simulink model "wheel_loader_dynamic"  (Simulink 8.3)
settings: Solver=ode45  StartTime=0.0  StopTime=8  RelTol=1e-3
values from neighbouring files (symbols this model uses):
  A_cylinder = pi * (r_pis^2 - r_rod^2)    [runSimLoader.m]
  c_fri_1 = 0.7196    [runSimLoader.m]
  c_fri_2 = -.01414    (= -0.01414)    [runSimLoader.m]
  c_fri_3 = 0.3590    (= 0.359)    [runSimLoader.m]
  c_p = 3e4    (= 30000)    [runSimLoader.m]
  c_p_m = [c_p1,c_p2,c_p3,c_p4]    [runSimLoader.m]
  c_r = 0.03    [runSimLoader.m]
  c_t1 = 38.5857    [runSimLoader.m]
  c_t2 = -0.6869    [runSimLoader.m]
  D_pump = 220/1900    (= 0.115789473684)    [runSimLoader.m]
  eta_gb = 0.9    [runSimLoader.m]
  eta_ig = 0.3623    [runSimLoader.m]
  eta_lift = 0.9    [runSimLoader.m]
  eta_vol_eng = 0.9    [runSimLoader.m]
  eta_volumetric = 0.98    [runSimLoader.m]
  gear_ratio = [-60 0 60]    [runSimLoader.m]
  I_ice = 3    [runSimLoader.m]
  k_theta = (diff(r .* sin(theta .* pi ./ 180)) ./ delta_theta)./ (div_delta_L)    [K_theta.m]
  M_boom = 5000    [runSimLoader.m]
  M_buc = 10000    [runSimLoader.m]
  M_load = 10000    [runSimLoader.m]
  M_veh = 32000    [runSimLoader.m]
  M_wheels = 4 .* J_w ./ r_w.^2    [runSimLoader.m]
  n_cyl = 6    [runSimLoader.m]
  n_cyl_hydra = 2    [runSimLoader.m]
  q_hv = 42.9e6    (= 42900000)    [runSimLoader.m]
  r = 2.9    [runSimLoader.m]
  r1 = 1.7    [runSimLoader.m]
  r_w = 0.7    [runSimLoader.m]
  Ra = 287    [runSimLoader.m]
  T_amb = 21 + 273.15    (= 294.15)    [runSimLoader.m]
  theta = -40:0.01:80    [runSimLoader.m]
  theta_1 = (atan((r1 * sin(theta .* pi ./ 180) - yc) ./ (r1 * cos(theta .* pi ./ 180 ) - xc))).* 180 ./ pi    [K_theta.m]
  u_str_max = 1 .* 180 ./ pi    [runSimLoader.m]
  u_str_min = -1 .* 180 ./ pi    [runSimLoader.m]
  Vd = 13e-3    (= 0.013)    [runSimLoader.m]
undefined symbols (not defined in the file or in its folder): sigbuilder_block
settings Model: Creator=beichuan  LastModifiedBy=beichuan
settings SolverCC: ZeroCrossControl=EnableAll
settings DataIOCC: SignalLoggingSaveFormat=Dataset
settings DebuggingCC: UnderspecifiedInitializationDetection=Simplified  MergeDetectMultiDrivingBlocksExec=error  FrameProcessingCompatibilityMsg=error  StateNameClashWarn=none
settings GRTTargetCC: CombineOutputUpdateFcns=on  GRTInterface=off

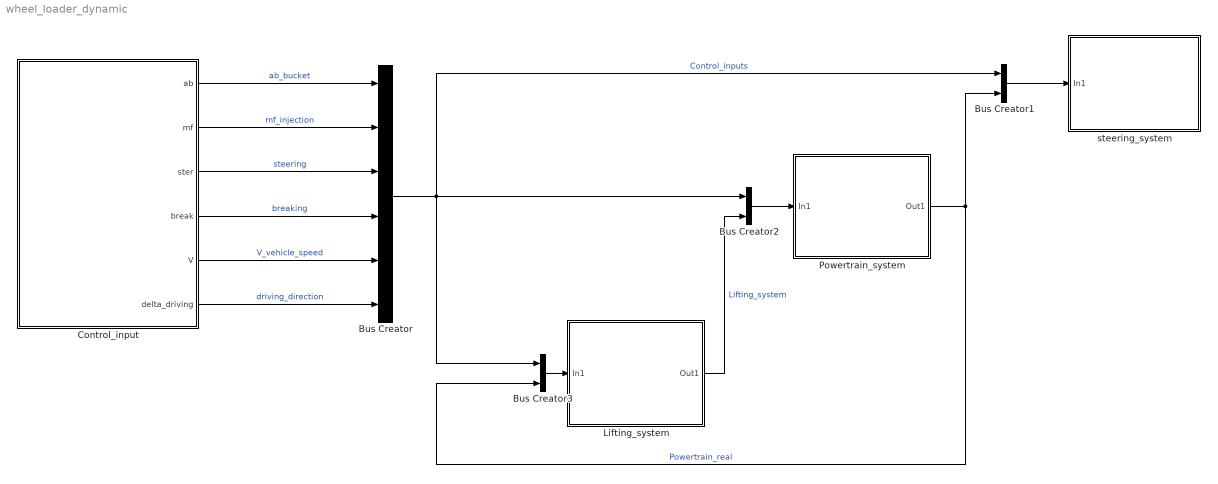
== system wheel_loader_dynamic ==
  Bus Creator : BusCreator  Inputs=6
  Bus Creator1 : BusCreator  Inputs=2
  Bus Creator2 : BusCreator  Inputs=2
  Bus Creator3 : BusCreator  Inputs=2
  Control_input : Subsystem  Tag=STV Subsys  LoadFcn=sigbuilder_block('load');  StartFcn=sigbuilder_block('start');  StopFcn=sigbuilder_block('stop');  ClipboardFcn=sigbuilder_block('clipboard');  mask(Sigbuilder block){}
      mask help: Simulink:masks:SigbuilderBlock_MD
      mask init:
      | if ~strcmp(get_param(bdroot(gcbh),'SimulationStatus'),'stopped') tuvar = sigbuilder_block('maskInit'); end
      settings: CopyFcn=sigbuilder_block('copy');  DeleteFcn=sigbuilder_block('delete');  ModelCloseFcn=sigbuilder_block('modelClose');  PreSaveFcn=sigbuilder_block('preSave');  PauseFcn=sigbuilder_block('pause');  ContinueFcn=sigbuilder_block('continue');  NameChangeFcn=sigbuilder_block('namechange');  OpenFcn=sigbuilder_block('open',[437.6 199.2 550.4 400 ]);  CloseFcn=sigbuilder_block('close');
      mask Display: plot(0, 0, 100, 100,[2, 2, 32, 32, 2], [68, 8, 8, 68, 68],[32, 2], [38, 38], [32, 19, 2],[53, 60, 44], [32, 17, 17, 2],[16, 16, 31, 31]);txt = getActiveGroup(gcbh);text(2, 100, txt,'verticalAlignment', 'top');
  Lifting_system : Subsystem
  Powertrain_system : Subsystem
  steering_system : Subsystem
  wires:
  Control_input/1(ab) -> Bus Creator/1  "ab_bucket"
  Control_input/2(mf) -> Bus Creator/2  "mf_injection"
  Control_input/3(ster) -> Bus Creator/3  "steering"
  Control_input/4(break) -> Bus Creator/4  "breaking"
  Control_input/5(V) -> Bus Creator/5  "V_vehicle_speed"
  Control_input/6(delta_driving) -> Bus Creator/6  "driving_direction"
  Bus Creator/1 -> Bus Creator3/1, Bus Creator2/1, Bus Creator1/1  "Control_inputs"
  Bus Creator1/1 -> steering_system/1(In1)
  Powertrain_system/1(Out1) -> Bus Creator3/2, Bus Creator1/2  "Powertrain_real"
  Lifting_system/1(Out1) -> Bus Creator2/2  "Lifting_system"
  Bus Creator2/1 -> Powertrain_system/1(In1)
  Bus Creator3/1 -> Lifting_system/1(In1)

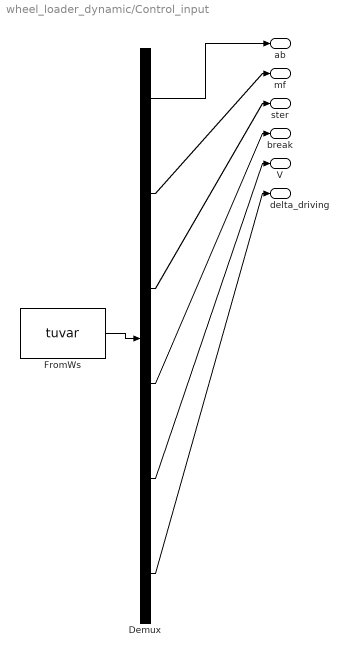
== system wheel_loader_dynamic/Control_input ==
  Demux : Demux  Tag=STV Demux  Outputs=6
  FromWs : FromWorkspace  Tag=STV FromWs  VariableName=tuvar  SampleTime=0  SigBuilderData=DataTag0  VnvData=DataTag1
      SigBuilderData=|
      | common.afterFinalStr = 'Extrapolate'
      | common.sampleTime = 0
      | dataSet.timeRange = [0 8]
      | dataSet.name = 'group1'
      | sbobj.Name = 'Signal Builder'
      | sbobj.Groups.Name = 'group1'
      | sbobj.Groups.Signals(1).Name = 'ab'
      | sbobj.Groups.Signals(1).XData = [0 0.1 0.2 0.3 0.4 0.5 0.6 0.7 0.8 0.9 1 1.1 1.2 1.3 1.4 1.5 1.6 1.7 1.8 1.9 2 2.1 2.2 2.3 2.4 2.5 2.6 2.7 2.8 2.9 3 3.1 3.2 3.3 3.4 3.5 3.6 3.7 3.8 3.9 4 4.1 4.2 4.3 4.4 4.5 4.6 4.7 4.8 4.9 5 5.1 5.2 5.3 5.4 5.5 5.6 5.7 5.8 5.9 6 6.1 6.2 6.3 6.4 6.5 6.6 6.7 6.8 6.9 7 7.1 7.2 7.3 7.4 7.5 7.6 7.7 7.8 7.9 8]
      | sbobj.Groups.Signals(1).YData = [0 0 0 0 0 0 0 0 0 0 0 0.0012 0.0037985136251 0.0308285163776 0.0706953932387 0.351412056152 0.609083402147 0.848224607762 0.935236522355 0.961161574456 0.976823561795 1.00066061107 1.05029294955 1.16939168731 1.3671345995 1.58238370493 1.60753096614 1.49205615194 1.22774566474 0.752127718139 0.227910817506 -0.265290393614 -0.852958987063 -1.50396366639 -1.99154968346 -2.30764290302 -2.40733278282 -2.35080282595 -2.09305807872 -1.59889898156 -0.765384210538 -0.178218185155 -0.0915606936416 -0.0498100743187 -0.0346820809249 -0.0338122763556 -0.0317240113772 -0.0277967834533 -0.0166096496402 -0.00100192678228 0.0428516377649 0.140379851363 0.450867052023 0.779741260666 1.05258935944 1.09202449766 1.07244701349 0.938356729975 0.756165703276 0.614958121977 0.461833195706 0.341701073493 0.326029911001 0.432832369942 0.61853014038 0.839187081384 0.934037985136 0.929967362668 0.763336085879 0.427250206441 -0.0169556840077 -0.531048720066 -0.987943848059 -1.42752546105 -1.83297550234 -2.02650701899 -2.04653637948 -1.88664097624 -1.6395045417 -1.08716396 -0.0666829688749]
      | sbobj.Groups.Signals(2).Name = 'mf'
      | sbobj.Groups.Signals(2).XData = [0 0.1 0.2 0.3 0.4 0.5 0.6 0.7 0.8 0.9 1 1.1 1.2 1.3 1.4 1.5 1.6 1.7 1.8 1.9 2 2.1 2.2 2.3 2.4 2.5 2.6 2.7 2.8 2.9 3 3.1 3.2 3.3 3.4 3.5 3.6 3.7 3.8 3.9 4 4.1 4.2 4.3 4.4 4.5 4.6 4.7 4.8 4.9 5 5.1 5.2 5.3 5.4 5.5 5.6 5.7 5.8 5.9 6 6.1 6.2 6.3 6.4 6.5 6.6 6.7 6.8 6.9 7 7.1 7.2 7.3 7.4 7.5 7.6 7.7 7.8 7.9 8]
      | sbobj.Groups.Signals(2).YData = [136.434293739 143.112254866 155.1515005 166.754707974 180.011757188 182.238887803 180.159590339 172.683073985 168.221152265 162.870442131 156.980918125 150.90837282 145.889314269 140.694401727 136.5035565 132.802576712 128.942985203 119.5157555 118.124919779 118.520007293 119.762934122 121.893233917 123.803492521 126.890630563 129.618601692 129.692037845 127.386820388 121.865342175 119.047224466 117.583964942 116.626273526 115.703766608 114.658502753 113.694665751 112.771263869 111.868612114 111.030017177 110.343726215 109.887048807 111.792247819 130.235850603 156.857423989 171.113363515 173.50521035 169.869285701 164.739623974 160.054532059 155.608792777 151.332202922 146.326683711 140.548059262 136.207910784 131.790419376 127.753572405 122.428802584 121.996378652 122.837925134 124.31155919 125.305409702 125.787848994 126.263185656 126.728874107 127.208296956 127.817096338 128.860663309 129.800113505 125.227927699 110.073892948 104.135933428 99.6392565962 94.9083453142 89.9787568932 84.4716215892 77.9962505896 72.6379264823 65.3454724982 56.6596769378 48.3989407366 40.9167034866 32.4113286548 23.3360227679]
      | sbobj.Groups.Signals(3).Name = 'ster'
      | sbobj.Groups.Signals(3).XData = [0 0.1 0.2 0.3 0.4 0.5 0.6 0.7 0.8 0.9 1 1.1 1.2 1.3 1.4 1.5 1.6 1.7 1.8 1.9 2 2.1 2.2 2.3 2.4 2.5 2.6 2.7 2.8 2.9 3 3.1 3.2 3.3 3.4 3.5 3.6 3.7 3.8 3.9 4 4.1 4.2 4.3 4.4 4.5 4.6 4.7 4.8 4.9 5 5.1 5.2 5.3 5.4 5.5 5.6 5.7 5.8 5.9 6 6.1 6.2 6.3 6.4 6.5 6.6 6.7 6.8 6.9 7 7.1 7.2 7.3 7.4 7.5 7.6 7.7 7.8 7.9 8]
      | sbobj.Groups.Signals(3).YData = [-0.0925407590775 -0.348691820217 -0.519811700234 -0.601650346981 -0.696257601694 -0.717202458972 -0.7078188363 -0.646098322879 -0.534483154388 -0.416420685048 -0.225672907369 -0.121565615644 -0.0359151364305 -0.0111173072785 -0.00135550773676 0.00195660035385 0.00206349260483 0.000951823699679 -0.000554343359518 -0.00201163482412 -0.0033936423166 -0.00421229854621 -0.00470911686372 -0.00493586432542 -0.0050357109239 -0.00371196745171 -0.00245082914425 -0.00157056884152 -0.00184308593844 -0.00274317825196 0.00153641501087 0.0546635806942 0.381728839487 0.781027336736 0.94506288199 0.972193776958 0.984213579311 0.990466350737 0.992225727179 0.992915876762 0.989741580163 0.975805930784 0.928989754399 0.723629422001 0.395948894451 0.0497204480852 -0.0186837459766 -0.0230294925796 -0.0235366519501 -0.0198871293351 -0.0171404101128 -0.016166285303 -0.0150270025514 -0.0149342113733 -0.0167159421425 -0.0190516599884 -0.0212529661437 -0.02310470684 -0.023982902125 -0.0248915932098 -0.0258587952054 -0.0260782650011 -0.0251671644417 -0.0243989390965 -0.0239285917259 -0.0234232137147 -0.0229493452476 -0.0260698680738 -0.0390836985518 -0.0916889465497 -0.21920578672 -0.412186632958 -0.581295933501 -0.700047433484 -0.771886573095 -0.785973823875 -0.760242512575 -0.687357288265 -0.542758632333 -0.338683697467 -0.0664566543993]
      | sbobj.Groups.Signals(4).Name = 'break'
      | sbobj.Groups.Signals(4).XData = [0 0.1 0.2 0.3 0.4 0.5 0.6 0.7 0.8 0.9 1 1.1 1.2 1.3 1.4 1.5 1.6 1.7 1.8 1.9 2 2.1 2.2 2.3 2.4 2.5 2.6 2.7 2.8 2.9 3 3.1 3.2 3.3 3.4 3.5 3.6 3.7 3.8 3.9 4 4.1 4.2 4.3 4.4 4.5 4.6 4.7 4.8 4.9 5 5.1 5.2 5.3 5.4 5.5 5.6 5.7 5.8 5.9 6 6.1 6.2 6.3 6.4 6.5 6.6 6.7 6.8 6.9 7 7.1 7.2 7.3 7.4 7.5 7.6 7.7 7.8 7.9 8]
      | sbobj.Groups.Signals(4).YData = [0 0 0 0 0 0 0 0 0 0 0 0 0 0 0 0 0 0 0 0 0 0 0 0 0 38000 38000 38000 38000 38000 38000 38000 38000 38000 38000 38000 38000 38000 38000 38000 38000 0 0 0 0 0 0 0 0 0 0 0 0 0 0 0 0 0 0 0 0 0 0 0 0 38000 38000 38000 38000 38000 38000 38000 38000 38000 38000 38000 38000 38000 38000 38000 38000]
      | sbobj.Groups.Signals(5).Name = 'V'
      | sbobj.Groups.Signals(5).XData = [0 0.1 0.2 0.3 0.4 0.5 0.6 0.7 0.8 0.9 1 1.1 1.2 1.3 1.4 1.5 1.6 1.7 1.8 1.9 2 2.1 2.2 2.3 2.4 2.5 2.6 2.7 2.8 2.9 3 3.1 3.2 3.3 3.4 3.5 3.6 3.7 3.8 3.9 4 4.1 4.2 4.3 4.4 4.5 4.6 4.7 4.8 4.9 5 5.1 5.2 5.3 5.4 5.5 5.6 5.7 5.8 5.9 6 6.1 6.2 6.3 6.4 6.5 6.6 6.7 6.8 6.9 7 7.1 7.2 7.3 7.4 7.5 7.6 7.7 7.8 7.9 8]
      | sbobj.Groups.Signals(5).YData = [0 -0.011853678733 -0.1489745147 -0.335139190768 -0.497249412755 -0.679980183949 -0.919070568803 -1.07507132247 -1.22614789893 -1.38144629545 -1.50859261387 -1.62060151025 -1.72478624892 -1.80801976225 -1.90153655881 -2.0214418959 -2.11077781921 -2.17353089181 -2.22833511797 -2.27846583683 -2.32219526667 -2.35987990242 -2.38573319504 -2.40624928505 -2.4109582345 -2.39480240961 -2.3574743765 -2.25843800036 -2.12607073756 -1.96315720809 -1.80420677077 -1.62248710194 -1.40291663121 -1.19787797702 -1.01826572769 -0.83573001019 -0.662802569374 -0.521012365637 -0.344334837653 -0.157996725109 0.0928254145755 0.419073303067 0.692563159034 0.911937970032 1.12247686448 1.25222430786 1.41064451903 1.55891157478 1.68954669623 1.79773195983 1.9248339803 1.99251547913 2.07003243768 2.1388410953 2.20100021744 2.2632567777 2.31372438824 2.34068037423 2.36349234459 2.3802368675 2.39179762706 2.40228292631 2.41359408091 2.42583884577 2.43136996862 2.42794234601 2.40275431012 2.35887488137 2.25945191937 2.06146439236 1.84202802708 1.69407702709 1.53714785936 1.3508089254 1.11068094692 0.97286033395 0.797666079222 0.593614863801 0.494193671774 0.358504813299 0.15468939199]
      | sbobj.Groups.Signals(6).Name = 'delta_driving'
      | sbobj.Groups.Signals(6).XData = [0 0.1 0.2 0.3 0.4 0.5 0.6 0.7 0.8 0.9 1 1.1 1.2 1.3 1.4 1.5 1.6 1.7 1.8 1.9 2 2.1 2.2 2.3 2.4 2.5 2.6 2.7 2.8 2.9 3 3.1 3.2 3.3 3.4 3.5 3.6 3.7 3.8 3.9 4 4.1 4.2 4.3 4.4 4.5 4.6 4.7 4.8 4.9 5 5.1 5.2 5.3 5.4 5.5 5.6 5.7 5.8 5.9 6 6.1 6.2 6.3 6.4 6.5 6.6 6.7 6.8 6.9 7 7.1 7.2 7.3 7.4 7.5 7.6 7.7 7.8 7.9 8]
      | sbobj.Groups.Signals(6).YData = [0 -0.843065657131 -2.04802634313 -3.67522211033 -5.13533975927 -7.16833788903 -9.4639006378 -11.2852477547 -12.6619084917 -14.0509869769 -15.4638584376 -16.1450583716 -16.4900313624 -16.7089519973 -16.7391055686 -16.7380195201 -16.7369334716 -16.7350386036 -16.7331523841 -16.7313534424 -16.7295545006 -16.7100313504 -16.6887416679 -16.6706223899 -16.655770768 -16.6409191462 -16.626305088 -16.6245590563 -16.6228130245 -16.4694711872 -16.2999050496 -15.7907008317 -14.8698900467 -13.2128172034 -11.0027054141 -9.01546731885 -6.52400134273 -3.5489397209 -0.430967246919 2.41629661599 4.93957703927 7.59207835803 10.2870139959 12.5207100897 14.3157512109 15.5236081139 16.0866296216 16.2456573994 16.4046851772 16.4710393389 16.4899987745 16.5089582101 16.5112570679 16.5125413392 16.5138256104 16.5152859936 16.516854621 16.5184293027 16.5201158107 16.5218023186 16.5420837638 16.5730794348 16.5913628987 16.6092910524 16.6255026455 16.6267195767 16.6279365079 16.6064875557 16.5486304129 16.49077327 15.9584731214 14.9941059526 13.670789239 11.9048865871 9.73122025608 7.66181844339 5.45443053757 3.66041960389 2.41178179227 1.31901381096 1]
      | sbobj.Groups.TimeRange = [0 8]
  ab : Outport
  mf : Outport  Tag=STV Outport  Port=2
  ster : Outport  Tag=STV Outport  Port=3
  break : Outport  Tag=STV Outport  Port=4
  V : Outport  Tag=STV Outport  Port=5
  delta_driving : Outport  Tag=STV Outport  Port=6
  wires:
  Demux/1 -> ab/1
  FromWs/1 -> Demux/1
  Demux/2 -> mf/1
  Demux/3 -> ster/1
  Demux/4 -> break/1
  Demux/5 -> V/1
  Demux/6 -> delta_driving/1

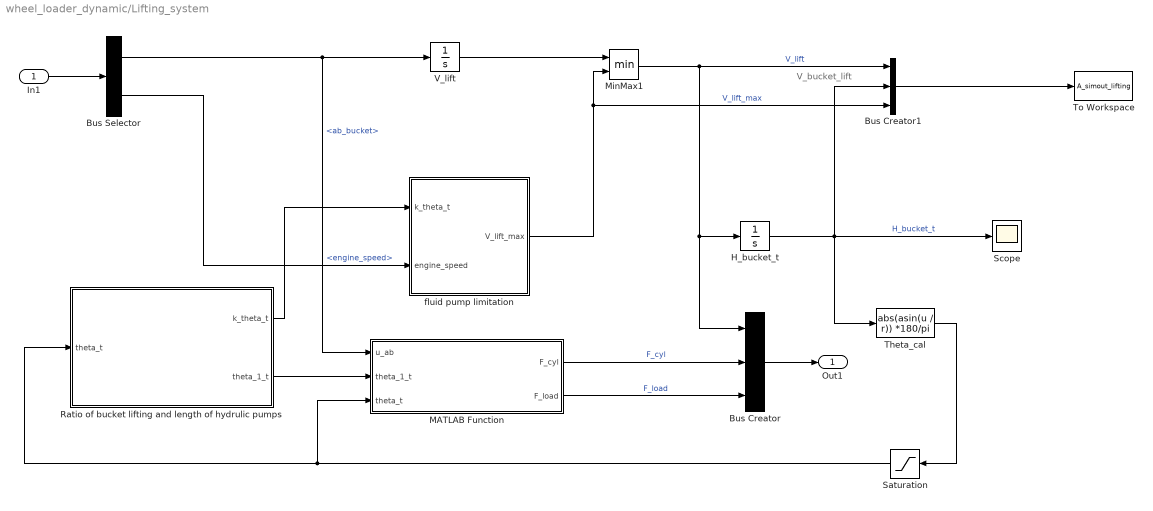
== system wheel_loader_dynamic/Lifting_system ==
  note: V_bucket_lift
  In1 : Inport
  Bus Creator : BusCreator  Inputs=3
  Bus Creator1 : BusCreator  Inputs=3
  Bus Selector : BusSelector  OutputSignals=Control_inputs.ab_bucket,Powertrain_real.engine_speed
  H_bucket_t : Integrator  InitialCondition=-0.9919
  MATLAB Function : MATLAB Function  TreatAsAtomicUnit=on
      settings: PermitHierarchicalResolution=ParametersOnly
  MinMax1 : MinMax  Inputs=2
  Ratio of bucket lifting and length of hydrulic pumps : MATLAB Function  TreatAsAtomicUnit=on
      settings: PermitHierarchicalResolution=ParametersOnly
  Saturation : Saturate  UpperLimit=max(theta)  LowerLimit=min(theta)
  Scope : Scope
      settings: TimeRange=auto  MaxDataPoints=5000  SaveToWorkspace=off  YMin=-1.48979  YMax=3.48909  SampleTime=-1
  Theta_cal : Fcn  Expr=abs(asin(u / r)) *180/pi
  To Workspace : ToWorkspace  VariableName=A_simout_lifting  SaveFormat=Structure With Time  SampleTime=-1
  V_lift : Integrator
  fluid pump limitation : MATLAB Function  TreatAsAtomicUnit=on
      settings: PermitHierarchicalResolution=ParametersOnly
  Out1 : Outport
  wires:
  In1/1 -> Bus Selector/1
  Bus Selector/1 -> V_lift/1, MATLAB Function/1(u_ab)  "<ab_bucket>"
  V_lift/1 -> MinMax1/1
  MinMax1/1 -> H_bucket_t/1, Bus Creator/1, Bus Creator1/1  "V_lift"
  H_bucket_t/1 -> Bus Creator1/2, Theta_cal/1, Scope/1  "H_bucket_t"
  Theta_cal/1 -> Saturation/1
  Ratio of bucket lifting and length of hydrulic pumps/2(theta_1_t) -> MATLAB Function/2(theta_1_t)
  Bus Creator/1 -> Out1/1
  Saturation/1 -> MATLAB Function/3(theta_t), Ratio of bucket lifting and length of hydrulic pumps/1(theta_t)
  Ratio of bucket lifting and length of hydrulic pumps/1(k_theta_t) -> fluid pump limitation/1(k_theta_t)
  MATLAB Function/1(F_cyl) -> Bus Creator/2  "F_cyl"
  MATLAB Function/2(F_load) -> Bus Creator/3  "F_load"
  Bus Selector/2 -> fluid pump limitation/2(engine_speed)  "<engine_speed>"
  fluid pump limitation/1(V_lift_max) -> Bus Creator1/3, MinMax1/2  "V_lift_max"
  Bus Creator1/1 -> To Workspace/1

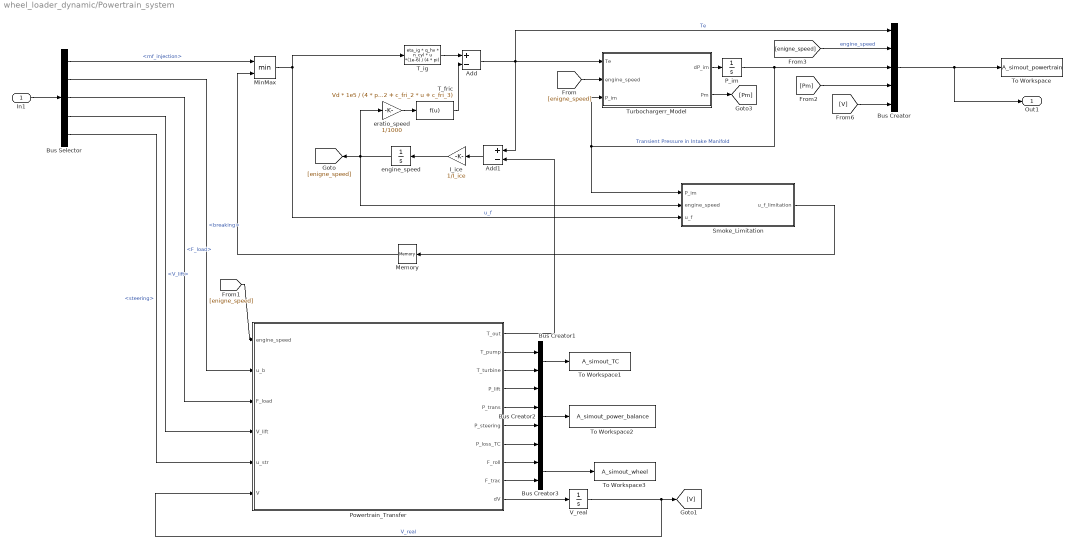
== system wheel_loader_dynamic/Powertrain_system ==
  In1 : Inport
  Add : Sum  Inputs=+-
  Add1 : Sum  Inputs=+-
  Bus Creator : BusCreator  Inputs=5
  Bus Creator1 : BusCreator  Inputs=2
  Bus Creator2 : BusCreator  Inputs=4
  Bus Creator3 : BusCreator  Inputs=2
  Bus Selector : BusSelector  OutputSignals=Control_inputs.mf_injection,Control_inputs.breaking,Lifting_system.F_load,Lifting_system.V_lift,Control_inputs.steering
  I_ice : Gain  Gain=1/I_ice
  Memory : Memory  X0=200
  MinMax : MinMax  Inputs=2
  P_im : Integrator  InitialCondition=1.3e5
  Powertrain_Transfer : MATLAB Function  TreatAsAtomicUnit=on
      settings: PermitHierarchicalResolution=ParametersOnly
  Smoke_Limitation : MATLAB Function  TreatAsAtomicUnit=on
      settings: PermitHierarchicalResolution=ParametersOnly
  T_fric : Fcn  Expr=Vd * 1e5 / (4 * pi) *(c_fri_1 * u^2 + c_fri_2 * u + c_fri_3)
  T_ig : Fcn  Expr=eta_ig * q_hv * n_cyl * u *(1e-6) / (4 * pi)
  To Workspace : ToWorkspace  VariableName=A_simout_powertrain  SaveFormat=Structure With Time  SampleTime=-1
  To Workspace1 : ToWorkspace  VariableName=A_simout_TC  SaveFormat=Structure With Time  SampleTime=-1
  To Workspace2 : ToWorkspace  VariableName=A_simout_power_balance  SaveFormat=Structure With Time  SampleTime=-1
  To Workspace3 : ToWorkspace  VariableName=A_simout_wheel  SaveFormat=Structure With Time  SampleTime=-1
  Turbochargerr_Model : MATLAB Function  TreatAsAtomicUnit=on
      settings: PermitHierarchicalResolution=ParametersOnly
  V_real : Integrator  InitialCondition=-0.02
  engine_speed : Integrator  InitialCondition=1432.4./60 .* 2 .* pi  LimitOutput=on  UpperSaturationLimit=230.38  LowerSaturationLimit=57
  eratio_speed : Gain  Gain=1/1000
  Out1 : Outport
  wires:
  In1/1 -> Bus Selector/1
  T_ig/1 -> Add/1
  T_fric/1 -> Add/2
  Add/1 -> Add1/1, Bus Creator/1, Turbochargerr_Model/1(Te)  "Te"
  Turbochargerr_Model/1(dP_im) -> P_im/1
  P_im/1 -> Bus Creator/3, Turbochargerr_Model/3(P_im), Smoke_Limitation/1(P_im)  "Transient Pressure in Intake Manifold"
  Bus Selector/1 -> MinMax/1  "<mf_injection>"
  Add1/1 -> I_ice/1
  MinMax/1 -> Smoke_Limitation/3(u_f), T_ig/1  "u_f"
  I_ice/1 -> engine_speed/1
  Powertrain_Transfer/1(T_out) -> Add1/2
  engine_speed/1 -> [enigne_speed], Smoke_Limitation/2(engine_speed), eratio_speed/1
  [enigne_speed] -> Turbochargerr_Model/2(engine_speed)
  [enigne_speed] -> Powertrain_Transfer/1(engine_speed)
  Powertrain_Transfer/10(dV) -> V_real/1
  V_real/1 -> [V], Powertrain_Transfer/6(V)  "V_real"
  Bus Creator/1 -> Out1/1, To Workspace/1
  Bus Selector/3 -> Powertrain_Transfer/3(F_load)  "<F_load>"
  eratio_speed/1 -> T_fric/1
  Bus Selector/4 -> Powertrain_Transfer/4(V_lift)  "<V_lift>"
  Bus Selector/5 -> Powertrain_Transfer/5(u_str)  "<steering>"
  Smoke_Limitation/1(u_f_limitation) -> Memory/1
  Memory/1 -> MinMax/2
  Turbochargerr_Model/2(Pm) -> [Pm]
  Bus Selector/2 -> Powertrain_Transfer/2(u_b)  "<breaking>"
  Bus Creator1/1 -> To Workspace1/1
  Powertrain_Transfer/2(T_pump) -> Bus Creator1/1
  Powertrain_Transfer/3(T_turbine) -> Bus Creator1/2
  [Pm] -> Bus Creator/4
  [V] -> Bus Creator/5
  [enigne_speed] -> Bus Creator/2  "engine_speed"
  Powertrain_Transfer/4(P_lift) -> Bus Creator2/1
  Powertrain_Transfer/5(P_trans) -> Bus Creator2/2
  Powertrain_Transfer/6(P_steering) -> Bus Creator2/3
  Powertrain_Transfer/7(P_loss_TC) -> Bus Creator2/4
  Bus Creator2/1 -> To Workspace2/1
  Powertrain_Transfer/8(F_roll) -> Bus Creator3/1
  Powertrain_Transfer/9(F_trac) -> Bus Creator3/2
  Bus Creator3/1 -> To Workspace3/1

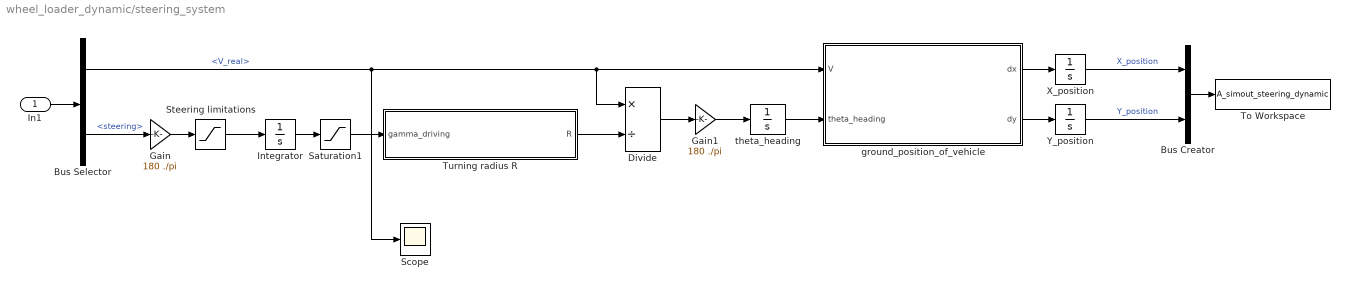
== system wheel_loader_dynamic/steering_system ==
  In1 : Inport
  Bus Creator : BusCreator  Inputs=2
  Bus Selector : BusSelector  OutputSignals=Powertrain_real.V_real,Control_inputs.steering
  Divide : Product  Inputs=*/
  Gain : Gain  Gain=180 ./pi
  Gain1 : Gain  Gain=180 ./pi
  Integrator : Integrator
  Saturation1 : Saturate  UpperLimit=20  LowerLimit=-20
  Scope : Scope
      settings: TimeRange=auto  MaxDataPoints=5000  SaveToWorkspace=off  YMin=-3.05154  YMax=2.61925  SampleTime=-1
  Steering limitations : Saturate  UpperLimit=u_str_max  LowerLimit=u_str_min
  To Workspace : ToWorkspace  VariableName=A_simout_steering_dynamic  SaveFormat=Structure With Time  SampleTime=-1
  Turning radius R : MATLAB Function  TreatAsAtomicUnit=on
      settings: PermitHierarchicalResolution=ParametersOnly
  X_position : Integrator  InitialCondition=25
  Y_position : Integrator  InitialCondition=40
  ground_position_of_vehicle : MATLAB Function  TreatAsAtomicUnit=on
      settings: PermitHierarchicalResolution=ParametersOnly
  theta_heading : Integrator  InitialCondition=90
  wires:
  In1/1 -> Bus Selector/1
  Bus Selector/2 -> Gain/1  "<steering>"
  Steering limitations/1 -> Integrator/1
  Integrator/1 -> Saturation1/1
  Saturation1/1 -> Turning radius R/1(gamma_driving)
  Turning radius R/1(R) -> Divide/2
  Bus Selector/1 -> Divide/1, ground_position_of_vehicle/1(V), Scope/1  "<V_real>"
  Divide/1 -> Gain1/1
  ground_position_of_vehicle/1(dx) -> X_position/1
  ground_position_of_vehicle/2(dy) -> Y_position/1
  X_position/1 -> Bus Creator/1  "X_position"
  Bus Creator/1 -> To Workspace/1
  Y_position/1 -> Bus Creator/2  "Y_position"
  Gain/1 -> Steering limitations/1
  Gain1/1 -> theta_heading/1
  theta_heading/1 -> ground_position_of_vehicle/2(theta_heading)

== matlab function steering_system/ground_position_of_vehicle ==
  data: V input double; dx output double; theta_heading input double; dy output double
function [dx,dy] = fcn(V,theta_heading)
%ground position of the vehicle: (x,y,theta)
dx = V .* cos(theta_heading .* pi ./ 180);
dy = V .* sin(theta_heading .* pi ./ 180);
end

== matlab function steering_system/Turning radius R ==
  data: gamma_driving input double; R output double
function R = fcn(gamma_driving)
% Turning radius R; unit: m
L = 3.7; %the length between the front and rear axles unit:m
R = L ./ (2 .* (tan((gamma_driving) .* 0.5 .* pi ./ 180)));
if ge(R,50)
    R = 50;
elseif le(R,-50)
    R = -50;
end

== matlab function Lifting_system/Ratio of bucket lifting and length of hydrulic pumps ==
  data: theta_t input double; k_theta_t output double; theta_1_t output double; theta_1 parameter double; k_theta parameter double; theta parameter double
function [k_theta_t,theta_1_t] = K_theta_finding(theta_t, theta_1, k_theta, theta)
%%% The lifting system 2014 version
%%% The Geometry coefficient of the lifting system
%%% k_theta is a ratio of bucket lifting and delta_length of hydrulic pumps
flag = 0;
k_theta_t = 10.56;
theta_1_t = 0;
for i = 1:length(theta)-1
    if (theta(i)<=theta_t) && (theta(i+1)>=theta_t)
        k_theta_t = 0.5 * (k_theta(i) + k_theta(i+1));
        theta_1_t = 0.5 * (theta_1(i) + theta_1(i+1));
        flag = 1;
        break
    end
end

if flag == 0
    k_theta_t = k_theta(end) ;
    theta_1_t =theta_1(end) ;
end

end

== matlab function Lifting_system/fluid pump limitation ==
  data: V_lift_max output double; k_theta_t input double; engine_speed input double; A_cylinder parameter double; D_pump parameter double; eta_volumetric parameter double; n_cyl_hydra parameter double
function V_lift_max  = fcn(k_theta_t, engine_speed, A_cylinder, D_pump, eta_volumetric, n_cyl_hydra)
% fluid pump limitation
% engine_speed = 1500./60; %unit: rps
% r_pis = 0.19./2; % radius of lift piston
% r_rod = 0.09./2; % radius of lift rod
% A_cylinder = pi * (r_pis^2 - r_rod^2);
% D_pump = 220/1900; % Hydraulic pump displacement
% eta_volumetric = 0.98; % Volumetric efficiency of the lift pump
% % eta_lift = 0.9; % efficiency of lift pump
% n_cyl_hydra = 2; % Cylider numbers of the hydratic system


Q_pump_max = min(engine_speed,157) .* D_pump .* eta_volumetric .* 10^-3;
v_cylinder_max = Q_pump_max .* n_cyl_hydra ./ A_cylinder;
V_lift_max = k_theta_t .* v_cylinder_max;

== matlab function Lifting_system/MATLAB Function ==
  data: u_ab input double; F_cyl output double; theta_1_t input double; theta_t input double; F_load output double; M_load parameter double; M_boom parameter double; r parameter double; r1 parameter double
function [F_cyl,F_load] = Force_cal(u_ab,theta_1_t,theta_t, M_load, M_boom, r, r1)
% Loading paremeters
% M_load = 10000; %the mass of loading; unit:kg
% M_boom = 5000; %the weight of the boom structure; unit:kg
% r = 2.9; % the boom length; 
% r1 = 1.7; % the boom length from body joint (O) to connection

F_cyl = ((M_boom .* 1.5 + M_load) * r * u_ab + (M_load + 0.5 .* M_boom) * 9.8 * r * cos(theta_t.* pi ./ 180)) ./ ...
    (r1 .* sin((theta_1_t - theta_t).* pi ./ 180));
F_load = M_load .* (9.8 + u_ab); % unit:N

== matlab function Powertrain_system/Turbochargerr_Model ==
  data: Te input double; dP_im output double; engine_speed input double; P_im input double; c_p_m parameter double; c_t1 parameter double; c_t2 parameter double; Pm output double
function [dP_im,Pm] = turbocharger(Te,engine_speed, P_im, c_p_m, c_t1, c_t2)
    %% the turbocharger system (1st order delay)
    Pm = c_p_m(1) .* (engine_speed).^2 + c_p_m(2) .* Te + c_p_m(4) .* (Te .* engine_speed) + c_p_m(3);
    Pm = Pm .* 4e-5;  % after 2 days guess, have to use a trick for controlling the value in the reasonable area.
    if ge(Pm , 4e5)
        Pm = 4e5;
    end
    tau_m = c_t1 .* (engine_speed).^c_t2;
    dP_im = 1 ./ tau_m .* (Pm - P_im);

== matlab function Powertrain_system/Smoke_Limitation ==
  data: P_im input double; engine_speed input double; u_f_limitation output double; u_f input double; eta_vol_eng parameter double; Vd parameter double; Ra parameter double; T_amb parameter double; n_cyl parameter double
function u_f_limitation  = somke_limitation(P_im, engine_speed, u_f, eta_vol_eng, Vd, Ra, T_amb, n_cyl)
%% the smoke limits
m_air = eta_vol_eng .* Vd .* engine_speed .* 60 ./ pi ./2 .* P_im ./ (4 .* pi .* Ra .* T_amb); % uint: kg/s
% m_f = 1e-6 ./ (4 .* pi) .* u_f .* engine_speed .* 60 ./ pi ./2 .* n_cyl; % unit: kg/s
u_f_limitation = 200;
lambda_minimum = 1.2; % the min of the air-fuel ratio;
if u_f ~= 0
    % lambda = ( m_air ./ m_f ) ./ 14.7; % 14.7 is the stoichiometric air to fuel ratio, and lambda is the air to fuel ratio indicator
    u_f_limitation = (m_air ./ (lambda_minimum .* 14.7)) ./ (1e-6 ./ (4 .* pi) .* engine_speed .* n_cyl .* 60 ./ pi ./2);
    
end

== matlab function Powertrain_system/Powertrain_Transfer ==
  data: engine_speed input double; u_b input double; F_load input double; V_lift input double; u_str input double; V input double; T_out output double; T_pump output double; T_turbine output double; P_lift output double; P_trans output double; P_steering output double; P_loss_TC output double; F_roll output double; F_trac output double; dV output double; eta_gb parameter double; c_r parameter double; c_p parameter double; M_veh parameter double; M_buc parameter double; M_wheels parameter double; r_w parameter double; gear_ratio parameter double; eta_lift parameter double
function [T_out,  T_pump, T_turbine , P_lift, P_trans, P_steering, P_loss_TC ,F_roll, F_trac , dV]   = powertrain( engine_speed, u_b, F_load, V_lift, u_str, V, eta_gb, c_r, c_p, M_veh, M_buc, M_wheels, r_w, gear_ratio, eta_lift)
%% vehicle powertrain system for moving
% the powertrain transfer
if sign(V) == 1
    gamma_gb = gear_ratio(3);
elseif sign(V) == -1
    gamma_gb = gear_ratio(1);
else
    gamma_gb = gear_ratio(2);
end
omega_gb = V .* gamma_gb ./ r_w;
Phi = omega_gb ./ engine_speed;

%% Torque converter
x = Phi;
p1 =      -57.24;  %(-107, -7.468)
p2 =        -177;  %(-479, 125)
p3 =        1339;  %(639.2, 2039)
p4 =       -1794;  %(-2566, -1022)
p5 =       334.3;  %(-75.2, 743.7)
p6 =      -39.47;  %(-131.2, 52.23)
p7 =       406.2;  %(400.1, 412.3)
ephsilon= p1*x^6 + p2*x^5 + p3*x^4 + p4*x^3 + p5*x^2 + p6*x + p7;

kappa_p1 =       26.26;%  (12.45, 40.06)
kappa_p2 =      -176.9;%  (-259.9, -93.83)
kappa_p3 =       427.4;%  (236.6, 618.1)
kappa_p4 =        -341;%  (-549.3, -132.8)
kappa_p5 =      -9.083;%  (-118.5, 100.3)
kappa_p6 =      -598.1;%  (-622.5, -573.7)
kappa_p7 =       675.4;%  (673.8, 677)
kappa = kappa_p1*x^6 + kappa_p2*x^5 + kappa_p3*x^4 + kappa_p4*x^3 + kappa_p5*x^2 + kappa_p6*x + kappa_p7;


%% output torque 
T_pump = ephsilon .* (engine_speed .*60 ./ (2 .* pi) ./1000).^2;
T_turbine = kappa .* (engine_speed .*60 ./ (2 .* pi) ./1000).^2;
T_w = T_turbine .* eta_gb .* gamma_gb;
% the vehicle moving
F_roll = sign(V) .* c_r .* (M_veh + M_buc) .* 9.8;
F_trac = (T_w - sign(V) .* u_b .* 1.66 ) ./ r_w; % the cofficient 1.66 is adopted for modification or I cannot get the result. This part is not right.
dV = (- F_roll  + F_trac ) ./ (M_buc + M_veh + M_wheels);

%% power balance for calculating the output torque
P_lift  = F_load  .* V_lift  ./ eta_lift; % unit:W
P_trans  = T_pump  .* engine_speed ;
P_steering  = (u_str).^2 .* c_p; % steering power; unit:W ./ 180 .* pi
T_out  = (P_trans  + P_steering  + P_lift )./ engine_speed ;
P_loss_TC = P_trans - T_turbine .*gamma_gb .* V ./r_w;
